simulink model "EstimadorFriccion"  (R2015a)
settings: Solver=ode45  StartTime=0.0  StopTime=40  RelTol=1e-3
libraries: simulink x1
settings Model: Creator=Usuario  LastModifiedBy=Usuario

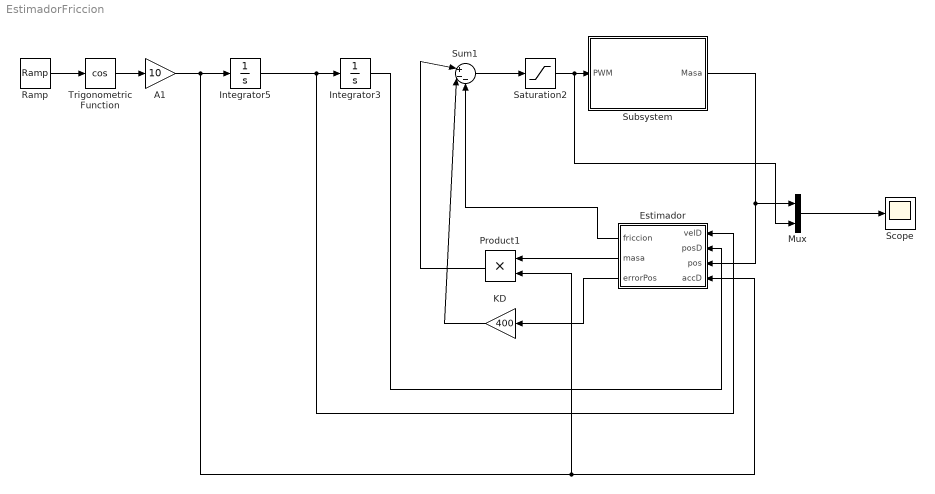
== system EstimadorFriccion ==
  A1 : Gain  Gain=10
  Estimador : Subsystem
  Integrator3 : Integrator
  Integrator5 : Integrator
  KD : Gain  Gain=400
  Mux : Mux  Inputs=2
  Product1 : Product
  Ramp : simulink/Sources/Ramp  slope=0.1  start=0  X0=0
  Saturation2 : Saturate  UpperLimit=100  LowerLimit=0
  Scope : Scope
      settings: TimeRange=10  YMin=0  YMax=2
  Subsystem : Subsystem
  Sum1 : Sum  Inputs=|+--
  Trigonometric Function : Trigonometry  Operator=cos
  wires:
  Integrator5/1 -> Estimador/1(velD), Integrator3/1
  Trigonometric Function/1 -> A1/1
  Subsystem/1(Masa) -> Mux/1, Estimador/3(pos)
  Estimador/2(masa) -> Product1/1
  Estimador/3(errorPos) -> KD/1
  Product1/1 -> Sum1/1
  KD/1 -> Sum1/2
  Estimador/1(friccion) -> Sum1/3
  Sum1/1 -> Saturation2/1
  Mux/1 -> Scope/1
  Ramp/1 -> Trigonometric Function/1
  Integrator3/1 -> Estimador/2(posD)
  A1/1 -> Product1/2, Estimador/4(accD), Integrator5/1
  Saturation2/1 -> Mux/2, Subsystem/1(PWM)

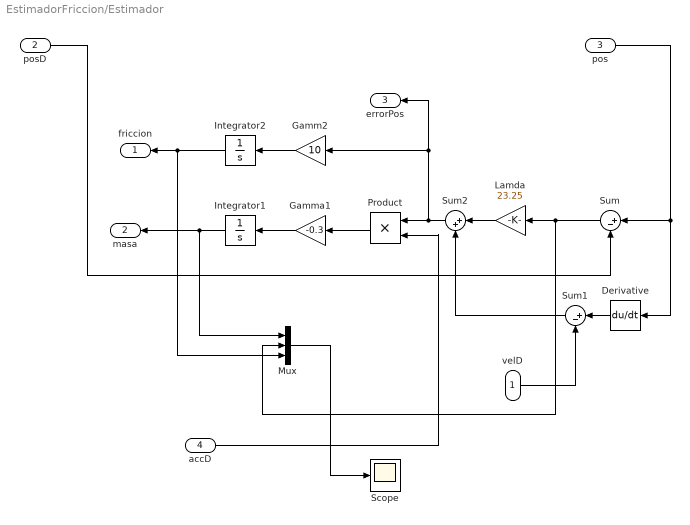
== system EstimadorFriccion/Estimador ==
  velD : Inport
  posD : Inport  Port=2
  pos : Inport  Port=3
  accD : Inport  Port=4
  Derivative : Derivative
  Gamm2 : Gain  Gain=10
  Gamma1 : Gain  Gain=-0.3
  Integrator1 : Integrator  InitialCondition=5.7
  Integrator2 : Integrator  InitialCondition=-10
  Lamda : Gain  Gain=23.25
  Mux : Mux  Inputs=3
  Product : Product
  Scope : Scope
  Sum : Sum  Inputs=|+-
  Sum1 : Sum  Inputs=|+-
  Sum2 : Sum  Inputs=|++
  friccion : Outport
  masa : Outport  Port=2
  errorPos : Outport  Port=3
  wires:
  posD/1 -> Sum/2
  Derivative/1 -> Sum1/1
  pos/1 -> Derivative/1, Sum/1
  Sum1/1 -> Sum2/2
  Gamm2/1 -> Integrator2/1
  accD/1 -> Product/2
  Integrator2/1 -> Mux/3, friccion/1
  Product/1 -> Gamma1/1
  Gamma1/1 -> Integrator1/1
  Sum2/1 -> errorPos/1, Gamm2/1, Product/1
  Integrator1/1 -> Mux/1, masa/1
  Lamda/1 -> Sum2/1
  Sum/1 -> Mux/2, Lamda/1
  velD/1 -> Sum1/2
  Mux/1 -> Scope/1

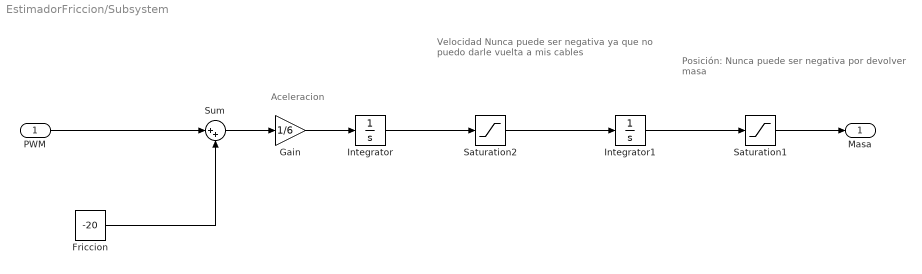
== system EstimadorFriccion/Subsystem ==
  note: Posición:
      | Nunca puede ser negativa por devolver masa
  note: Velocidad
      | Nunca puede ser negativa ya que no puedo
      | darle vuelta a mis cables
  note: Aceleracion
  PWM : Inport
  Friccion : Constant  Value=-20
  Gain : Gain  Gain=1/6
  Integrator : Integrator
  Integrator1 : Integrator
  Saturation1 : Saturate  UpperLimit=100000  LowerLimit=0
  Saturation2 : Saturate  UpperLimit=100000  LowerLimit=0
  Sum : Sum  Inputs=|++
  Masa : Outport
  wires:
  Integrator1/1 -> Saturation1/1
  Integrator/1 -> Saturation2/1
  Saturation1/1 -> Masa/1
  Gain/1 -> Integrator/1
  Sum/1 -> Gain/1
  PWM/1 -> Sum/1
  Friccion/1 -> Sum/2
  Saturation2/1 -> Integrator1/1
